simulink model "MGietka_4"  (R2020b)
settings: Solver=VariableStepAuto  StartTime=0.0  StopTime=10.0  RelTol=1e-3
undefined symbols (not defined in the file): A, B, C, K, L, N
libraries: simulink x1
settings Model: Creator=Mati  LastModifiedBy=Mati

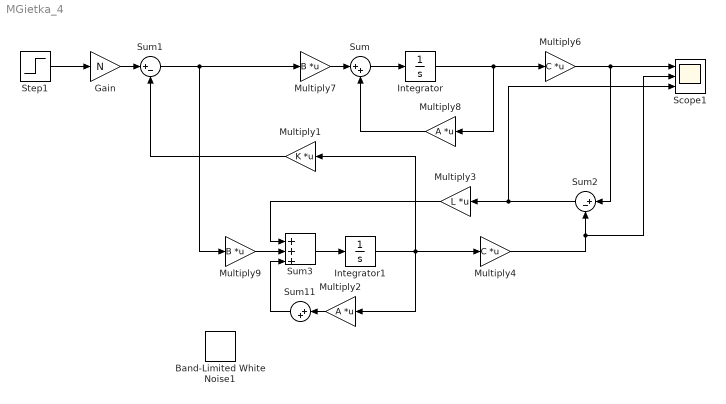
== system MGietka_4 ==
  Band-Limited White Noise1 : simulink/Sources/Band-Limited White Noise  Cov=[0.0001]  Ts=0.1  seed=[23341]
  Gain : Gain  Gain=N
  Integrator : Integrator
  Integrator1 : Integrator
  Multiply1 : Gain  Gain=K  Multiplication=Matrix(K*u)
  Multiply2 : Gain  Gain=A  Multiplication=Matrix(K*u)
  Multiply3 : Gain  Gain=L  Multiplication=Matrix(K*u)
  Multiply4 : Gain  Gain=C  Multiplication=Matrix(K*u)
  Multiply6 : Gain  Gain=C  Multiplication=Matrix(K*u)
  Multiply7 : Gain  Gain=B  Multiplication=Matrix(K*u)
  Multiply8 : Gain  Gain=A  Multiplication=Matrix(K*u)
  Multiply9 : Gain  Gain=B  Multiplication=Matrix(K*u)
  Scope1 : Scope  NumInputPorts=3
  Step1 : Step  SampleTime=0
  Sum : Sum  Inputs=|++
  Sum1 : Sum  Inputs=|+-
  Sum11 : Sum  Inputs=|++
  Sum2 : Sum  Inputs=|+-
  Sum3 : Sum  Inputs=|+|+|+
  wires:
  Multiply4/1 -> Sum2/2, Scope1/2
  Multiply8/1 -> Sum/2
  Sum1/1 -> Multiply7/1, Multiply9/1
  Multiply9/1 -> Sum3/2
  Sum3/1 -> Integrator1/1
  Multiply7/1 -> Sum/1
  Step1/1 -> Gain/1
  Integrator/1 -> Multiply6/1, Multiply8/1
  Multiply6/1 -> Scope1/1, Sum2/1
  Sum2/1 -> Scope1/3, Multiply3/1
  Gain/1 -> Sum1/1
  Integrator1/1 -> Multiply2/1, Multiply4/1, Multiply1/1
  Sum/1 -> Integrator/1
  Multiply1/1 -> Sum1/2
  Multiply2/1 -> Sum11/1
  Sum11/1 -> Sum3/3
  Multiply3/1 -> Sum3/1
